simulink model "BBeva2"  (R2020a)
settings: Solver=ode23  StartTime=0.0  StopTime=30  RelTol=1e-6  AbsTol=1e-6  EnableMultiTasking=on
InitFcn:
  | beta = 0.002;
  | g = 9.81;
  | x0 = 10;
  | mu = 0.9;
settings Model: ExtModeAutoUpdateStatusClock=off  Creator=peter  LastModifiedBy=peter
settings DataIOCC: LimitDataPoints=on  SaveFormat=Array  SignalLoggingSaveFormat=ModelDataLogs  ReturnWorkspaceOutputs=off  SignalLoggingName=sigsOut  Refine=10
settings OptimizationCC: BooleanDataType=off  ExpressionDepthLimit=2147483647  LifeSpan=inf
settings DebuggingCC: AlgebraicLoopMsg=none  SaveWithParameterizedLinksMsg=none  UnderspecifiedInitializationDetection=Classic  MergeDetectMultiDrivingBlocksExec=none  SignalResolutionControl=TryResolveAllWithWarning  MultiTaskDSMMsg=warning  MultiTaskCondExecSysMsg=none  FcnCallInpInsideContextMsg=warning  StateNameClashWarn=warning  SFUnexpectedBacktrackingDiag=warning  SFNoUnconditionalDefaultTransitionDiag=warning  SFExecutionAtInitializationDiag=none  ArithmeticOperatorsInVariantConditions=warning
settings HardwareCC: ProdBitPerPointer=32  ProdBitPerSizeT=32  ProdBitPerPtrDiffT=32  ProdLargestAtomicFloat=None  ProdIntDivRoundTo=Undefined  ProdEndianess=Unspecified  ProdWordSize=32  ProdHWDeviceType=32-bit Generic  TargetUnknown=on
settings ModelReferenceCC: PropagateSignalLabelsOutOfModel=off
settings SFSimCC: SimUseLocalCustomCode=off  CustomCodeUndefinedFunction=UseInterfaceOnly
settings RTWCC: RTWUseLocalCustomCode=off
settings CodeAppCC: StateflowObjectComments=on
settings GRTTargetCC: TargetLangStandard=C89/C90 (ANSI)  CombineOutputUpdateFcns=off  GRTInterface=on
settings ConfigComp: CovMetricSettings=dw  CovHtmlReporting=on  CovSaveCumulativeToWorkspaceVar=on  CovSaveSingleToWorkspaceVar=on  CovExternalEMLEnable=off

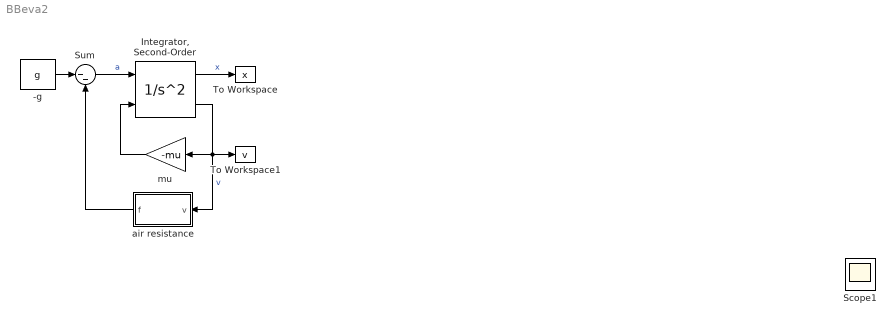
== system BBeva2 ==
  -g : Constant  Value=g
  "Integrator, Second-Order" : SecondOrderIntegrator  ICX=x0  LimitX=on  LowerLimitX=0  ICSourceDXDT=external  ReinitDXDTwhenXreachesSaturation=on
  Sum : Sum  Inputs=|--
  To Workspace : ToWorkspace  VariableName=x  SaveFormat=Timeseries  SampleTime=-1
  To Workspace1 : ToWorkspace  VariableName=v  SaveFormat=Timeseries  SampleTime=-1
  air resistance : Subsystem  mask{beta=beta}
  mu : Gain  Gain=-mu  SaturateOnIntegerOverflow=on  OutDataTypeStr=Inherit: Same as input  ParamDataTypeStr=Inherit: Same as input
  Scope1 : Scope
  wires:
  "Integrator, Second-Order"/2 -> air resistance/1(v), To Workspace1/1, mu/1  "v"
  "Integrator, Second-Order"/1 -> To Workspace/1  "x"
  mu/1 -> "Integrator, Second-Order"/2
  Sum/1 -> "Integrator, Second-Order"/1  "a"
  -g/1 -> Sum/1
  air resistance/1(f) -> Sum/2

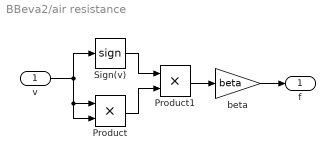
== system BBeva2/air resistance ==
  v : Inport
  Product : Product
  Product1 : Product
  Sign(v) : Signum
  beta : Gain  Gain=beta
  f : Outport
  wires:
  v/1 -> Sign(v)/1, Product/2, Product/1
  Product/1 -> Product1/2
  Sign(v)/1 -> Product1/1
  Product1/1 -> beta/1
  beta/1 -> f/1
